simulink model "W01_Base_World_real_time_cs"  (R2019a)
settings: Solver=FixedStepDiscrete  StartTime=0.0  StopTime=100  FixedStep=1/10  RelTol=1e-3
PreLoadFcn:
  | mbxruntime.callbacks.PreLoadFcn(bdroot);
  | check_NUTS_defined
  | model_closed = 0;
  | assignin('base',['model_closed_' bdroot],false);
PostLoadFcn:
  | mbxruntime.callbacks.PostLoadFcn(bdroot);
InitFcn:
  | mbxruntime.callbacks.InitFcn(bdroot);
StartFcn:
  | mbxruntime.callbacks.StartFcn(bdroot);
StopFcn:
  | mbxruntime.callbacks.StopFcn(bdroot);;
  | 
model workspace: external: MAT-File .\W01_Base_World_real_time_cs_hws.mat (data not in the file)
undefined symbols (not defined in the file): DiscIntNeverNeededParam, Header, InitImageOutputDir, mbxruntime, Orientation, Poses, Poses_SL_Info, Position, tabledata, W01_Base_World_real_time_cs_0b088fecc0986594, W01_Base_World_real_time_cs_1aae0b63dd3ae7f4, W01_Base_World_real_time_cs_220fcdeecd830796, W01_Base_World_real_time_cs_3877e8e14bce73ac, W01_Base_World_real_time_cs_4300902b6df2ef4f, W01_Base_World_real_time_cs_4b27c2527ab847ef, W01_Base_World_real_time_cs_5a21cbbf439ca820, W01_Base_World_real_time_cs_5fa564e8c61193e5, W01_Base_World_real_time_cs_830b936d13a49cea, W01_Base_World_real_time_cs_930ade6322553a76, W01_Base_World_real_time_cs_ac8882985e6a0180, W01_Base_World_real_time_cs_ae21d31eb95a5608, W01_Base_World_real_time_cs_Audi_A8_Sedan_1_Path_pathUniqueID, W01_Base_World_real_time_cs_b246a85ce45846f9, W01_Base_World_real_time_cs_b2518551f2cbcab1, W01_Base_World_real_time_cs_b7bc831679541a88, W01_Base_World_real_time_cs_dae62575d56496ac, W01_Base_World_real_time_cs_de41d194e5862055, W01_Base_World_real_time_cs_Male_RegularAni_1_Path_pathUniqueID, W01_Base_World_real_time_cs_Male_RegularAni_2_Path_pathUniqueID
libraries: adeye_lib x37, simulink_extras x30, simulink x10, robotlib x4, sharedtransform x2, PreScanSimulinkLibrary x2
(part 4 of 8)

== system W01_Base_World_real_time_cs/PreScanTerminator ==
  Terminator : Terminator
  sfun_Terminator : S-Function  FunctionName=sfun_Terminator  Parameters=SampleTime  SFunctionDeploymentMode=off  EnableBusSupport=off  mask(Legacy Function){SFunctionSpec=void prescan_terminator_outputFcn(void ** work1, PRESCAN_TERMINATORDATA y1[1]), SampleTime=TimeStep, ShowSpec=on}
      mask prompts: SampleTime "Sample time (-1 for inherited):"; ShowSpec "Display function specification"
      mask help:
      | This block allows you to call the legacy functions specified by the following Legacy Code Tool definition:
      | def.SFunctionName = 'sfun_Terminator';
      | def.OutputFcnSpec = 'void prescan_terminator_outputFcn(void ** work1, PRESCAN_TERMINATORDATA y1[1])';
      | def.StartFcnSpec = 'void prescan_terminator_startFcn(void ** work1)';
      | def.TerminateFcnSpec = 'void prescan_terminator_terminateFcn(void ** work1)';
      | def.HeaderFiles = {'prescan_terminator_data.h'};
      | def.HostLibFiles = {'sensorinterfaced.lib'};
      | def.IncPaths = {'src', 'C:\prescandev\vislibrary\vis\..\pimp\include\sensors\InterfaceRTW'};
      | def.SrcPaths = {'src'};
      | def.LibPaths = {'C:\\prescandev\\vislibrary_build\lib'};
      | def.SampleTime = 'parameterized';
      | def.Options.language = 'C';
      mask Help: <p>This block was generated automatically by the Legacy Code Tool. For detailed help on this tool, call<a href="matlab:legacy_code('help')"> legacy_code('help')</a>.</p>
      mask Callback ShowSpec:
      | if strcmp(get_param(gcbh, 'ShowSpec'), 'on')
      |   set_param(gcbh, 'MaskDisplay', sprintf('fprintf(''%s'');', get_param(gcbh, 'SFunctionSpec')));
      | else
      |   set_param(gcbh, 'MaskDisplay', sprintf('fprintf(''%s'');', get_param(gcbh, 'FunctionName')));
      | end
      mask Display: fprintf('void prescan_terminator_outputFcn(void ** work1, PRESCAN_TERMINATORDATA y1[1])');
  wires:
  sfun_Terminator/1 -> Terminator/1

== system W01_Base_World_real_time_cs/SELF_Audi_A8_Sedan_1 ==
  Sensor : S-Function  FunctionName=sfun_SelfSensor  Parameters=mbxruntime.parameters.convert(UniqueID), mbxruntime.parameters.convert(TimeStep)  SFunctionDeploymentMode=off  EnableBusSupport=off  mask(PreScan Source Block: SELF){UniqueID=18645, TimeStep=1/10}
      mask prompts: UniqueID "Auto-Assigned: Unique ID"; TimeStep "Auto-Assigned: Upload Period [s]"
      mask help:
      | The SELF port shows (state) information of the actor itself. The outputs are position in the experiment's axis system and the GPS coordinates, and the object's absolute velocity and compass heading.
      |
      | For more information, please click Help.
      mask Help: eval('openHelp(462)')
      mask Display: image(imread('GPS.png'))
  SELF_Audi_A8_Sedan_1 : Outport  Tag=outport/SelfPort  OutDataTypeStr=Bus: PRESCAN_SELFSENSORDATA  PortDimensions=1  SampleTime=1/10
  wires:
  Sensor/1 -> SELF_Audi_A8_Sedan_1/1

== system W01_Base_World_real_time_cs/SELF_BMW_X5_SUV_1 ==
  Sensor : S-Function  FunctionName=sfun_SelfSensor  Parameters=mbxruntime.parameters.convert(UniqueID), mbxruntime.parameters.convert(TimeStep)  SFunctionDeploymentMode=off  EnableBusSupport=off  mask(PreScan Source Block: SELF){UniqueID=9040, TimeStep=1/10}
      mask prompts: UniqueID "Auto-Assigned: Unique ID"; TimeStep "Auto-Assigned: Upload Period [s]"
      mask help:
      | The SELF port shows (state) information of the actor itself. The outputs are position in the experiment's axis system and the GPS coordinates, and the object's absolute velocity and compass heading.
      |
      | For more information, please click Help.
      mask Help: eval('openHelp(462)')
      mask Display: image(imread('GPS.png'))
  SELF_BMW_X5_SUV_1 : Outport  Tag=outport/SelfPort  OutDataTypeStr=Bus: PRESCAN_SELFSENSORDATA  PortDimensions=1  SampleTime=1/10
  wires:
  Sensor/1 -> SELF_BMW_X5_SUV_1/1

== system W01_Base_World_real_time_cs/SELF_Child_RegularAni_1 ==
  Sensor : S-Function  FunctionName=sfun_SelfSensor  Parameters=mbxruntime.parameters.convert(UniqueID), mbxruntime.parameters.convert(TimeStep)  SFunctionDeploymentMode=off  EnableBusSupport=off  mask(PreScan Source Block: SELF){UniqueID=18395, TimeStep=1/10}
      mask prompts: UniqueID "Auto-Assigned: Unique ID"; TimeStep "Auto-Assigned: Upload Period [s]"
      mask help:
      | The SELF port shows (state) information of the actor itself. The outputs are position in the experiment's axis system and the GPS coordinates, and the object's absolute velocity and compass heading.
      |
      | For more information, please click Help.
      mask Help: eval('openHelp(462)')
      mask Display: image(imread('GPS.png'))
  SELF_Child_RegularAni_1 : Outport  Tag=outport/SelfPort  OutDataTypeStr=Bus: PRESCAN_SELFSENSORDATA  PortDimensions=1  SampleTime=1/10
  wires:
  Sensor/1 -> SELF_Child_RegularAni_1/1

== system W01_Base_World_real_time_cs/SELF_Child_RegularAni_2 ==
  Sensor : S-Function  FunctionName=sfun_SelfSensor  Parameters=mbxruntime.parameters.convert(UniqueID), mbxruntime.parameters.convert(TimeStep)  SFunctionDeploymentMode=off  EnableBusSupport=off  mask(PreScan Source Block: SELF){UniqueID=18628, TimeStep=1/10}
      mask prompts: UniqueID "Auto-Assigned: Unique ID"; TimeStep "Auto-Assigned: Upload Period [s]"
      mask help:
      | The SELF port shows (state) information of the actor itself. The outputs are position in the experiment's axis system and the GPS coordinates, and the object's absolute velocity and compass heading.
      |
      | For more information, please click Help.
      mask Help: eval('openHelp(462)')
      mask Display: image(imread('GPS.png'))
  SELF_Child_RegularAni_2 : Outport  Tag=outport/SelfPort  OutDataTypeStr=Bus: PRESCAN_SELFSENSORDATA  PortDimensions=1  SampleTime=1/10
  wires:
  Sensor/1 -> SELF_Child_RegularAni_2/1

== system W01_Base_World_real_time_cs/SELF_Citroen_C3_Hatchback_1 ==
  Sensor : S-Function  FunctionName=sfun_SelfSensor  Parameters=mbxruntime.parameters.convert(UniqueID), mbxruntime.parameters.convert(TimeStep)  SFunctionDeploymentMode=off  EnableBusSupport=off  mask(PreScan Source Block: SELF){UniqueID=18857, TimeStep=1/10}
      mask prompts: UniqueID "Auto-Assigned: Unique ID"; TimeStep "Auto-Assigned: Upload Period [s]"
      mask help:
      | The SELF port shows (state) information of the actor itself. The outputs are position in the experiment's axis system and the GPS coordinates, and the object's absolute velocity and compass heading.
      |
      | For more information, please click Help.
      mask Help: eval('openHelp(462)')
      mask Display: image(imread('GPS.png'))
  SELF_Citroen_C3_Hatchback_1 : Outport  Tag=outport/SelfPort  OutDataTypeStr=Bus: PRESCAN_SELFSENSORDATA  PortDimensions=1  SampleTime=1/10
  wires:
  Sensor/1 -> SELF_Citroen_C3_Hatchback_1/1

== system W01_Base_World_real_time_cs/SELF_Female_RegularAni_1 ==
  Sensor : S-Function  FunctionName=sfun_SelfSensor  Parameters=mbxruntime.parameters.convert(UniqueID), mbxruntime.parameters.convert(TimeStep)  SFunctionDeploymentMode=off  EnableBusSupport=off  mask(PreScan Source Block: SELF){UniqueID=18631, TimeStep=1/10}
      mask prompts: UniqueID "Auto-Assigned: Unique ID"; TimeStep "Auto-Assigned: Upload Period [s]"
      mask help:
      | The SELF port shows (state) information of the actor itself. The outputs are position in the experiment's axis system and the GPS coordinates, and the object's absolute velocity and compass heading.
      |
      | For more information, please click Help.
      mask Help: eval('openHelp(462)')
      mask Display: image(imread('GPS.png'))
  SELF_Female_RegularAni_1 : Outport  Tag=outport/SelfPort  OutDataTypeStr=Bus: PRESCAN_SELFSENSORDATA  PortDimensions=1  SampleTime=1/10
  wires:
  Sensor/1 -> SELF_Female_RegularAni_1/1

== system W01_Base_World_real_time_cs/SELF_Male_RegularAni_1 ==
  Sensor : S-Function  FunctionName=sfun_SelfSensor  Parameters=mbxruntime.parameters.convert(UniqueID), mbxruntime.parameters.convert(TimeStep)  SFunctionDeploymentMode=off  EnableBusSupport=off  mask(PreScan Source Block: SELF){UniqueID=18634, TimeStep=1/10}
      mask prompts: UniqueID "Auto-Assigned: Unique ID"; TimeStep "Auto-Assigned: Upload Period [s]"
      mask help:
      | The SELF port shows (state) information of the actor itself. The outputs are position in the experiment's axis system and the GPS coordinates, and the object's absolute velocity and compass heading.
      |
      | For more information, please click Help.
      mask Help: eval('openHelp(462)')
      mask Display: image(imread('GPS.png'))
  SELF_Male_RegularAni_1 : Outport  Tag=outport/SelfPort  OutDataTypeStr=Bus: PRESCAN_SELFSENSORDATA  PortDimensions=1  SampleTime=1/10
  wires:
  Sensor/1 -> SELF_Male_RegularAni_1/1

== system W01_Base_World_real_time_cs/SELF_Male_RegularAni_2 ==
  Sensor : S-Function  FunctionName=sfun_SelfSensor  Parameters=mbxruntime.parameters.convert(UniqueID), mbxruntime.parameters.convert(TimeStep)  SFunctionDeploymentMode=off  EnableBusSupport=off  mask(PreScan Source Block: SELF){UniqueID=18853, TimeStep=1/10}
      mask prompts: UniqueID "Auto-Assigned: Unique ID"; TimeStep "Auto-Assigned: Upload Period [s]"
      mask help:
      | The SELF port shows (state) information of the actor itself. The outputs are position in the experiment's axis system and the GPS coordinates, and the object's absolute velocity and compass heading.
      |
      | For more information, please click Help.
      mask Help: eval('openHelp(462)')
      mask Display: image(imread('GPS.png'))
  SELF_Male_RegularAni_2 : Outport  Tag=outport/SelfPort  OutDataTypeStr=Bus: PRESCAN_SELFSENSORDATA  PortDimensions=1  SampleTime=1/10
  wires:
  Sensor/1 -> SELF_Male_RegularAni_2/1

== system W01_Base_World_real_time_cs/STATE_Audi_A8_Sedan_1_bus ==
  STATE_Audi_A8_Sedan_1_bus : Inport  Tag=inport/StatePort  OutDataTypeStr=Bus: PRESCAN_STATEACTUATORDATA  PortDimensions=1  SampleTime=1/10  BusOutputAsStruct=on
  Actuator : S-Function  FunctionName=sfun_StateActuator  Parameters=mbxruntime.parameters.convert(UniqueID), mbxruntime.parameters.convert(TimeStep)  SFunctionDeploymentMode=off  EnableBusSupport=off  mask(PreScan Sink Block: State){UniqueID=18645, TimeStep=1/10}
      mask prompts: UniqueID "Auto-Assigned: Unique ID"; TimeStep "Auto-Assigned: Upload Period [s]"
      mask help:
      | The Actor State contains a vector signal of size (9x1), containing the following signals:
      |
      | -  Position    	(x,y,z)             	[m]
      | -  Velocity    	(vx,vy,vz)         	[m/s]
      | -  Angles       	(Roll, Pitch, Yaw)	[rad]
      |
      | The Actor state is defined in the global axis system.
      | The state is superponed on the Initial position defined in the GUI.
      |
      | For more information, please click Help.
      mask Help: eval('openHelp(222)')
      mask Display: image(imread('State.png'))
  wires:
  STATE_Audi_A8_Sedan_1_bus/1 -> Actuator/1

== system W01_Base_World_real_time_cs/STATE_BMW_X5_SUV_1_bus ==
  STATE_BMW_X5_SUV_1_bus : Inport  Tag=inport/StatePort  OutDataTypeStr=Bus: PRESCAN_STATEACTUATORDATA  PortDimensions=1  SampleTime=1/10  BusOutputAsStruct=on
  Actuator : S-Function  FunctionName=sfun_StateActuator  Parameters=mbxruntime.parameters.convert(UniqueID), mbxruntime.parameters.convert(TimeStep)  SFunctionDeploymentMode=off  EnableBusSupport=off  mask(PreScan Sink Block: State){UniqueID=9040, TimeStep=1/10}
      mask prompts: UniqueID "Auto-Assigned: Unique ID"; TimeStep "Auto-Assigned: Upload Period [s]"
      mask help:
      | The Actor State contains a vector signal of size (9x1), containing the following signals:
      |
      | -  Position    	(x,y,z)             	[m]
      | -  Velocity    	(vx,vy,vz)         	[m/s]
      | -  Angles       	(Roll, Pitch, Yaw)	[rad]
      |
      | The Actor state is defined in the global axis system.
      | The state is superponed on the Initial position defined in the GUI.
      |
      | For more information, please click Help.
      mask Help: eval('openHelp(222)')
      mask Display: image(imread('State.png'))
  wires:
  STATE_BMW_X5_SUV_1_bus/1 -> Actuator/1

== system W01_Base_World_real_time_cs/STATE_Child_RegularAni_1_bus ==
  STATE_Child_RegularAni_1_bus : Inport  Tag=inport/StatePort  OutDataTypeStr=Bus: PRESCAN_STATEACTUATORDATA  PortDimensions=1  SampleTime=1/10  BusOutputAsStruct=on
  Actuator : S-Function  FunctionName=sfun_StateActuator  Parameters=mbxruntime.parameters.convert(UniqueID), mbxruntime.parameters.convert(TimeStep)  SFunctionDeploymentMode=off  EnableBusSupport=off  mask(PreScan Sink Block: State){UniqueID=18395, TimeStep=1/10}
      mask prompts: UniqueID "Auto-Assigned: Unique ID"; TimeStep "Auto-Assigned: Upload Period [s]"
      mask help:
      | The Actor State contains a vector signal of size (9x1), containing the following signals:
      |
      | -  Position    	(x,y,z)             	[m]
      | -  Velocity    	(vx,vy,vz)         	[m/s]
      | -  Angles       	(Roll, Pitch, Yaw)	[rad]
      |
      | The Actor state is defined in the global axis system.
      | The state is superponed on the Initial position defined in the GUI.
      |
      | For more information, please click Help.
      mask Help: eval('openHelp(222)')
      mask Display: image(imread('State.png'))
  wires:
  STATE_Child_RegularAni_1_bus/1 -> Actuator/1

== system W01_Base_World_real_time_cs/STATE_Child_RegularAni_2_bus ==
  STATE_Child_RegularAni_2_bus : Inport  Tag=inport/StatePort  OutDataTypeStr=Bus: PRESCAN_STATEACTUATORDATA  PortDimensions=1  SampleTime=1/10  BusOutputAsStruct=on
  Actuator : S-Function  FunctionName=sfun_StateActuator  Parameters=mbxruntime.parameters.convert(UniqueID), mbxruntime.parameters.convert(TimeStep)  SFunctionDeploymentMode=off  EnableBusSupport=off  mask(PreScan Sink Block: State){UniqueID=18628, TimeStep=1/10}
      mask prompts: UniqueID "Auto-Assigned: Unique ID"; TimeStep "Auto-Assigned: Upload Period [s]"
      mask help:
      | The Actor State contains a vector signal of size (9x1), containing the following signals:
      |
      | -  Position    	(x,y,z)             	[m]
      | -  Velocity    	(vx,vy,vz)         	[m/s]
      | -  Angles       	(Roll, Pitch, Yaw)	[rad]
      |
      | The Actor state is defined in the global axis system.
      | The state is superponed on the Initial position defined in the GUI.
      |
      | For more information, please click Help.
      mask Help: eval('openHelp(222)')
      mask Display: image(imread('State.png'))
  wires:
  STATE_Child_RegularAni_2_bus/1 -> Actuator/1

== system W01_Base_World_real_time_cs/STATE_Citroen_C3_Hatchback_1_bus ==
  STATE_Citroen_C3_Hatchback_1_bus : Inport  Tag=inport/StatePort  OutDataTypeStr=Bus: PRESCAN_STATEACTUATORDATA  PortDimensions=1  SampleTime=1/10  BusOutputAsStruct=on
  Actuator : S-Function  FunctionName=sfun_StateActuator  Parameters=mbxruntime.parameters.convert(UniqueID), mbxruntime.parameters.convert(TimeStep)  SFunctionDeploymentMode=off  EnableBusSupport=off  mask(PreScan Sink Block: State){UniqueID=18857, TimeStep=1/10}
      mask prompts: UniqueID "Auto-Assigned: Unique ID"; TimeStep "Auto-Assigned: Upload Period [s]"
      mask help:
      | The Actor State contains a vector signal of size (9x1), containing the following signals:
      |
      | -  Position    	(x,y,z)             	[m]
      | -  Velocity    	(vx,vy,vz)         	[m/s]
      | -  Angles       	(Roll, Pitch, Yaw)	[rad]
      |
      | The Actor state is defined in the global axis system.
      | The state is superponed on the Initial position defined in the GUI.
      |
      | For more information, please click Help.
      mask Help: eval('openHelp(222)')
      mask Display: image(imread('State.png'))
  wires:
  STATE_Citroen_C3_Hatchback_1_bus/1 -> Actuator/1

== system W01_Base_World_real_time_cs/STATE_Female_RegularAni_1_bus ==
  STATE_Female_RegularAni_1_bus : Inport  Tag=inport/StatePort  OutDataTypeStr=Bus: PRESCAN_STATEACTUATORDATA  PortDimensions=1  SampleTime=1/10  BusOutputAsStruct=on
  Actuator : S-Function  FunctionName=sfun_StateActuator  Parameters=mbxruntime.parameters.convert(UniqueID), mbxruntime.parameters.convert(TimeStep)  SFunctionDeploymentMode=off  EnableBusSupport=off  mask(PreScan Sink Block: State){UniqueID=18631, TimeStep=1/10}
      mask prompts: UniqueID "Auto-Assigned: Unique ID"; TimeStep "Auto-Assigned: Upload Period [s]"
      mask help:
      | The Actor State contains a vector signal of size (9x1), containing the following signals:
      |
      | -  Position    	(x,y,z)             	[m]
      | -  Velocity    	(vx,vy,vz)         	[m/s]
      | -  Angles       	(Roll, Pitch, Yaw)	[rad]
      |
      | The Actor state is defined in the global axis system.
      | The state is superponed on the Initial position defined in the GUI.
      |
      | For more information, please click Help.
      mask Help: eval('openHelp(222)')
      mask Display: image(imread('State.png'))
  wires:
  STATE_Female_RegularAni_1_bus/1 -> Actuator/1

== system W01_Base_World_real_time_cs/STATE_Male_RegularAni_1_bus ==
  STATE_Male_RegularAni_1_bus : Inport  Tag=inport/StatePort  OutDataTypeStr=Bus: PRESCAN_STATEACTUATORDATA  PortDimensions=1  SampleTime=1/10  BusOutputAsStruct=on
  Actuator : S-Function  FunctionName=sfun_StateActuator  Parameters=mbxruntime.parameters.convert(UniqueID), mbxruntime.parameters.convert(TimeStep)  SFunctionDeploymentMode=off  EnableBusSupport=off  mask(PreScan Sink Block: State){UniqueID=18634, TimeStep=1/10}
      mask prompts: UniqueID "Auto-Assigned: Unique ID"; TimeStep "Auto-Assigned: Upload Period [s]"
      mask help:
      | The Actor State contains a vector signal of size (9x1), containing the following signals:
      |
      | -  Position    	(x,y,z)             	[m]
      | -  Velocity    	(vx,vy,vz)         	[m/s]
      | -  Angles       	(Roll, Pitch, Yaw)	[rad]
      |
      | The Actor state is defined in the global axis system.
      | The state is superponed on the Initial position defined in the GUI.
      |
      | For more information, please click Help.
      mask Help: eval('openHelp(222)')
      mask Display: image(imread('State.png'))
  wires:
  STATE_Male_RegularAni_1_bus/1 -> Actuator/1

== system W01_Base_World_real_time_cs/STATE_Male_RegularAni_2_bus ==
  STATE_Male_RegularAni_2_bus : Inport  Tag=inport/StatePort  OutDataTypeStr=Bus: PRESCAN_STATEACTUATORDATA  PortDimensions=1  SampleTime=1/10  BusOutputAsStruct=on
  Actuator : S-Function  FunctionName=sfun_StateActuator  Parameters=mbxruntime.parameters.convert(UniqueID), mbxruntime.parameters.convert(TimeStep)  SFunctionDeploymentMode=off  EnableBusSupport=off  mask(PreScan Sink Block: State){UniqueID=18853, TimeStep=1/10}
      mask prompts: UniqueID "Auto-Assigned: Unique ID"; TimeStep "Auto-Assigned: Upload Period [s]"
      mask help:
      | The Actor State contains a vector signal of size (9x1), containing the following signals:
      |
      | -  Position    	(x,y,z)             	[m]
      | -  Velocity    	(vx,vy,vz)         	[m/s]
      | -  Angles       	(Roll, Pitch, Yaw)	[rad]
      |
      | The Actor state is defined in the global axis system.
      | The state is superponed on the Initial position defined in the GUI.
      |
      | For more information, please click Help.
      mask Help: eval('openHelp(222)')
      mask Display: image(imread('State.png'))
  wires:
  STATE_Male_RegularAni_2_bus/1 -> Actuator/1

== system W01_Base_World_real_time_cs/ScenarioEngine ==
  Clock : Clock
  sfun_ScenarioEngine : S-Function  FunctionName=sfun_ScenarioEngine  Parameters=TimeStep  SFunctionDeploymentMode=off  EnableBusSupport=off
  wires:
  Clock/1 -> sfun_ScenarioEngine/1

== system W01_Base_World_real_time_cs/Synchronizer ==
  Bus Selector1 : BusSelector  OutputSignals=FederateStopped
  Stop Simulation : Stop
  sfun_Synchronizer : S-Function  FunctionName=sfun_Synchronizer  Parameters=SampleTime  SFunctionDeploymentMode=off  EnableBusSupport=off  mask(Legacy Function){SFunctionSpec=void prescan_synchronizer_outputFcn(void ** work1, PRESCAN_SYNCHRONIZEDATA y1[1]), SampleTime=TimeStep, ShowSpec=on}
      mask prompts: SampleTime "Sample time (-1 for inherited):"; ShowSpec "Display function specification"
      mask help:
      | This block allows you to call the legacy functions specified by the following Legacy Code Tool definition:
      | def.SFunctionName = 'sfun_Synchronizer';
      | def.OutputFcnSpec = 'void prescan_synchronizer_outputFcn(void ** work1, PRESCAN_TIMESTAMPDATA u1[1], PRESCAN_SYNCHRONIZEDATA y1[1])';
      | def.StartFcnSpec = 'void prescan_synchronizer_startFcn(void ** work1)';
      | def.TerminateFcnSpec = 'void prescan_synchronizer_terminateFcn(void ** work1)';
      | def.HeaderFiles = {'prescan_synchronizer_data.h'};
      | def.HostLibFiles = {'sensorinterfaced.lib'};
      | def.IncPaths = {'src', 'C:\prescandev\vislibrary\vis\..\pimp\include\sensors\InterfaceRTW'};
      | def.SrcPaths = {'src'};
      | def.LibPaths = {'C:\\prescandev\\vislibrary_build\lib'};
      | def.SampleTime = 'parameterized';
      | def.Options.language = 'C';
      mask Help: <p>This block was generated automatically by the Legacy Code Tool. For detailed help on this tool, call<a href="matlab:legacy_code('help')"> legacy_code('help')</a>.</p>
      mask Callback ShowSpec:
      | if strcmp(get_param(gcbh, 'ShowSpec'), 'on')
      |   set_param(gcbh, 'MaskDisplay', sprintf('fprintf(''%s'');', get_param(gcbh, 'SFunctionSpec')));
      | else
      |   set_param(gcbh, 'MaskDisplay', sprintf('fprintf(''%s'');', get_param(gcbh, 'FunctionName')));
      | end
      mask Display: fprintf('void prescan_synchronizer_outputFcn(void ** work1, PRESCAN_SYNCHRONIZEDATA y1[1])');
  wires:
  sfun_Synchronizer/1 -> Bus Selector1/1
  Bus Selector1/1 -> Stop Simulation/1  "<FederateStopped>"

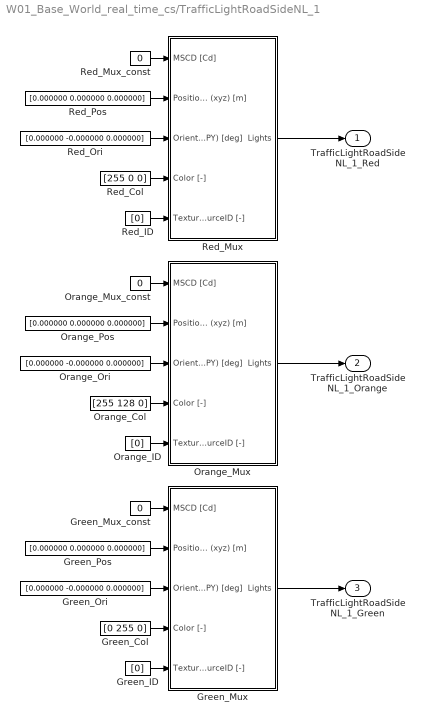
== system W01_Base_World_real_time_cs/TrafficLightRoadSideNL_1 ==
  Green_Col : Constant  Tag=VisuLightConst  Value=[0 255 0]
  Green_ID : Constant  Tag=VisuLightConst  Value=[0]
  Green_Mux : Subsystem  Tag=mux/ActiveLight  mask(PreScan User Interface: VisuActiveLight){}
      mask help:
      | The VisuActiveLight block provides a way for detailed animation of Light Sources, such as the indicator, brake, fog and main lights of a vehicle, or a light post.
      |
      | For more information, please click Help.
      settings: DeleteFcn=PreScanBlockDeleteFcn;
      mask Help: eval('openHelp(209)')
  Green_Mux_const : Constant  Tag=VisuLightConst  Value=0
  Green_Ori : Constant  Tag=VisuLightConst  Value=[0.000000 -0.000000 0.000000]
  Green_Pos : Constant  Tag=VisuLightConst  Value=[0.000000 0.000000 0.000000]
  Orange_Col : Constant  Tag=VisuLightConst  Value=[255 128 0]
  Orange_ID : Constant  Tag=VisuLightConst  Value=[0]
  Orange_Mux : Subsystem  Tag=mux/ActiveLight  mask(PreScan User Interface: VisuActiveLight){}
      mask help:
      | The VisuActiveLight block provides a way for detailed animation of Light Sources, such as the indicator, brake, fog and main lights of a vehicle, or a light post.
      |
      | For more information, please click Help.
      settings: DeleteFcn=PreScanBlockDeleteFcn;
      mask Help: eval('openHelp(209)')
  Orange_Mux_const : Constant  Tag=VisuLightConst  Value=0
  Orange_Ori : Constant  Tag=VisuLightConst  Value=[0.000000 -0.000000 0.000000]
  Orange_Pos : Constant  Tag=VisuLightConst  Value=[0.000000 0.000000 0.000000]
  Red_Col : Constant  Tag=VisuLightConst  Value=[255 0 0]
  Red_ID : Constant  Tag=VisuLightConst  Value=[0]
  Red_Mux : Subsystem  Tag=mux/ActiveLight  mask(PreScan User Interface: VisuActiveLight){}
      mask help:
      | The VisuActiveLight block provides a way for detailed animation of Light Sources, such as the indicator, brake, fog and main lights of a vehicle, or a light post.
      |
      | For more information, please click Help.
      settings: DeleteFcn=PreScanBlockDeleteFcn;
      mask Help: eval('openHelp(209)')
  Red_Mux_const : Constant  Tag=VisuLightConst  Value=0
  Red_Ori : Constant  Tag=VisuLightConst  Value=[0.000000 -0.000000 0.000000]
  Red_Pos : Constant  Tag=VisuLightConst  Value=[0.000000 0.000000 0.000000]
  TrafficLightRoadSideNL_1_Red : Outport  Tag=outport/Red  OutDataTypeStr=Bus: PRESCAN_VISULIGHTACTUATOR_DATA  SampleTime=1/10
  TrafficLightRoadSideNL_1_Orange : Outport  Tag=outport/Orange  Port=2  OutDataTypeStr=Bus: PRESCAN_VISULIGHTACTUATOR_DATA  SampleTime=1/10
  TrafficLightRoadSideNL_1_Green : Outport  Tag=outport/Green  Port=3  OutDataTypeStr=Bus: PRESCAN_VISULIGHTACTUATOR_DATA  SampleTime=1/10
  wires:
  Green_Mux_const/1 -> Green_Mux/1(MSCD [Cd])
  Orange_Mux_const/1 -> Orange_Mux/1(MSCD [Cd])
  Red_Mux_const/1 -> Red_Mux/1(MSCD [Cd])
  Red_Mux/1(Lights) -> TrafficLightRoadSideNL_1_Red/1
  Red_Pos/1 -> Red_Mux/2(Position (xyz) [m])
  Red_Ori/1 -> Red_Mux/3(Orientation (RPY) [deg])
  Red_Col/1 -> Red_Mux/4(Color [-])
  Red_ID/1 -> Red_Mux/5(TextureResourceID [-])
  Orange_Mux/1(Lights) -> TrafficLightRoadSideNL_1_Orange/1
  Orange_Pos/1 -> Orange_Mux/2(Position (xyz) [m])
  Orange_Ori/1 -> Orange_Mux/3(Orientation (RPY) [deg])
  Orange_Col/1 -> Orange_Mux/4(Color [-])
  Orange_ID/1 -> Orange_Mux/5(TextureResourceID [-])
  Green_Mux/1(Lights) -> TrafficLightRoadSideNL_1_Green/1
  Green_Pos/1 -> Green_Mux/2(Position (xyz) [m])
  Green_Ori/1 -> Green_Mux/3(Orientation (RPY) [deg])
  Green_Col/1 -> Green_Mux/4(Color [-])
  Green_ID/1 -> Green_Mux/5(TextureResourceID [-])

== system W01_Base_World_real_time_cs/TrafficLightRoadSideNL_1_Green ==
  TrafficLightRoadSideNL_1_Green : Inport  Tag=inport/Green  OutDataTypeStr=Bus: PRESCAN_VISULIGHTACTUATOR_DATA  SampleTime=1/10  BusOutputAsStruct=on
  Actuator : S-Function  FunctionName=sfun_VisuLightActuator  Parameters=mbxruntime.parameters.convert(UniqueID), mbxruntime.parameters.convert(LightName), mbxruntime.parameters.convert(PivotName), mbxruntime.parameters.convert(TextureResources), mbxruntime.parameters.convert(ColorsObjectName), mbxruntime.parameters.convert(MeshOnColor), mbxruntime.parameters.convert(MeshOffColor), tabledata, TimeStep  SFunctionDeploymentMode=off  EnableBusSupport=off  mask(PreScan Sink Block: VisuActiveLight){UniqueID=646, LightName=TrafficLightRoadSideNL_1.LightActuator_2_Green_ActiveLight, PivotName=TrafficLightRoadSideNL_1.Green, TextureResources={ 'Resources/LightMap/GeneralLight.png'}, ColorsObjectName=TrafficLightRoadSideNL_1.Green, MeshOnColor=[0  100    0  255    0  100    0  255  102  102  102  255    0  510    0  255], MeshOffColor=[0  100    0  255    0  100    0  255  102  102  102  255    0    0    0  255], TimeStep=1/10}
      mask prompts: UniqueID "Parent Unique Identifier"; LightName "Light"; PivotName "Pivot"; TextureResources "Texture Resources"; ColorsObjectName "Light Fixture Color Object"; MeshOnColor "Light Fixture On Color"; MeshOffColor "Light Fixture Off Color"; TimeStep "Simulink time step"
      mask help:
      | The VisuActiveLight block provides a way for detailed animation of Light Sources, such as the indicator, brake, fog and main lights of a vehicle, or a light post.
      |
      | For more information, please click Help.
      mask init:
      | [tabledata] = mbxruntime.parameters.table(UniqueID,LightName,PivotName,TextureResources,ColorsObjectName,MeshOnColor,MeshOffColor);
      mask Help: eval('openHelp(209)')
      mask Display: image(imread('HeadLight.png'))
  wires:
  TrafficLightRoadSideNL_1_Green/1 -> Actuator/1

== system W01_Base_World_real_time_cs/TrafficLightRoadSideNL_1_Orange ==
  TrafficLightRoadSideNL_1_Orange : Inport  Tag=inport/Orange  OutDataTypeStr=Bus: PRESCAN_VISULIGHTACTUATOR_DATA  SampleTime=1/10  BusOutputAsStruct=on
  Actuator : S-Function  FunctionName=sfun_VisuLightActuator  Parameters=mbxruntime.parameters.convert(UniqueID), mbxruntime.parameters.convert(LightName), mbxruntime.parameters.convert(PivotName), mbxruntime.parameters.convert(TextureResources), mbxruntime.parameters.convert(ColorsObjectName), mbxruntime.parameters.convert(MeshOnColor), mbxruntime.parameters.convert(MeshOffColor), tabledata, TimeStep  SFunctionDeploymentMode=off  EnableBusSupport=off  mask(PreScan Sink Block: VisuActiveLight){UniqueID=646, LightName=TrafficLightRoadSideNL_1.LightActuator_1_Orange_ActiveLight, PivotName=TrafficLightRoadSideNL_1.Orange, TextureResources={ 'Resources/LightMap/GeneralLight.png'}, ColorsObjectName=TrafficLightRoadSideNL_1.Orange, MeshOnColor=[100   50    0  255  100   50    0  255  102  102  102  255  510  256    0  255], MeshOffColor=[100   50    0  255  100   50    0  255  102  102  102  255    0    0    0  255], TimeStep=1/10}
      mask prompts: UniqueID "Parent Unique Identifier"; LightName "Light"; PivotName "Pivot"; TextureResources "Texture Resources"; ColorsObjectName "Light Fixture Color Object"; MeshOnColor "Light Fixture On Color"; MeshOffColor "Light Fixture Off Color"; TimeStep "Simulink time step"
      mask help:
      | The VisuActiveLight block provides a way for detailed animation of Light Sources, such as the indicator, brake, fog and main lights of a vehicle, or a light post.
      |
      | For more information, please click Help.
      mask init:
      | [tabledata] = mbxruntime.parameters.table(UniqueID,LightName,PivotName,TextureResources,ColorsObjectName,MeshOnColor,MeshOffColor);
      mask Help: eval('openHelp(209)')
      mask Display: image(imread('HeadLight.png'))
  wires:
  TrafficLightRoadSideNL_1_Orange/1 -> Actuator/1

== system W01_Base_World_real_time_cs/TrafficLightRoadSideNL_1_Red ==
  TrafficLightRoadSideNL_1_Red : Inport  Tag=inport/Red  OutDataTypeStr=Bus: PRESCAN_VISULIGHTACTUATOR_DATA  SampleTime=1/10  BusOutputAsStruct=on
  Actuator : S-Function  FunctionName=sfun_VisuLightActuator  Parameters=mbxruntime.parameters.convert(UniqueID), mbxruntime.parameters.convert(LightName), mbxruntime.parameters.convert(PivotName), mbxruntime.parameters.convert(TextureResources), mbxruntime.parameters.convert(ColorsObjectName), mbxruntime.parameters.convert(MeshOnColor), mbxruntime.parameters.convert(MeshOffColor), tabledata, TimeStep  SFunctionDeploymentMode=off  EnableBusSupport=off  mask(PreScan Sink Block: VisuActiveLight){UniqueID=646, LightName=TrafficLightRoadSideNL_1.LightActuator_0_Red_ActiveLight, PivotName=TrafficLightRoadSideNL_1.Red, TextureResources={ 'Resources/LightMap/GeneralLight.png'}, ColorsObjectName=TrafficLightRoadSideNL_1.Red, MeshOnColor=[100    0    0  255  100    0    0  255  102  102  102  255  510    0    0  255], MeshOffColor=[100    0    0  255  100    0    0  255  102  102  102  255    0    0    0  255], TimeStep=1/10}
      mask prompts: UniqueID "Parent Unique Identifier"; LightName "Light"; PivotName "Pivot"; TextureResources "Texture Resources"; ColorsObjectName "Light Fixture Color Object"; MeshOnColor "Light Fixture On Color"; MeshOffColor "Light Fixture Off Color"; TimeStep "Simulink time step"
      mask help:
      | The VisuActiveLight block provides a way for detailed animation of Light Sources, such as the indicator, brake, fog and main lights of a vehicle, or a light post.
      |
      | For more information, please click Help.
      mask init:
      | [tabledata] = mbxruntime.parameters.table(UniqueID,LightName,PivotName,TextureResources,ColorsObjectName,MeshOnColor,MeshOffColor);
      mask Help: eval('openHelp(209)')
      mask Display: image(imread('HeadLight.png'))
  wires:
  TrafficLightRoadSideNL_1_Red/1 -> Actuator/1

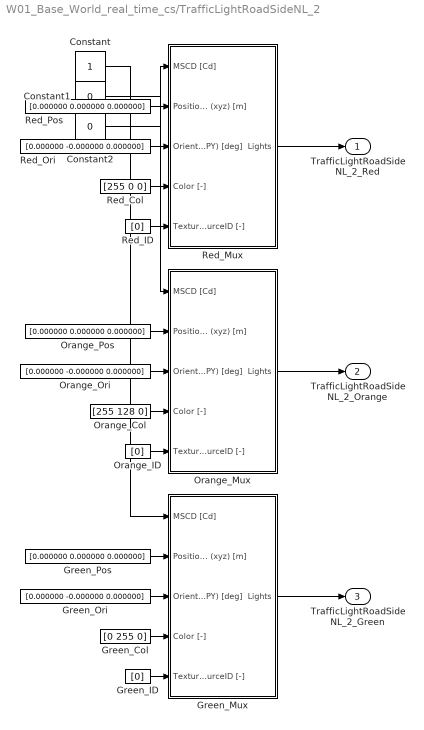
== system W01_Base_World_real_time_cs/TrafficLightRoadSideNL_2 ==
  Constant : Constant
  Constant1 : Constant  Value=0
  Constant2 : Constant  Value=0
  Green_Col : Constant  Tag=VisuLightConst  Value=[0 255 0]
  Green_ID : Constant  Tag=VisuLightConst  Value=[0]
  Green_Mux : Subsystem  Tag=mux/ActiveLight  mask(PreScan User Interface: VisuActiveLight){}
      mask help:
      | The VisuActiveLight block provides a way for detailed animation of Light Sources, such as the indicator, brake, fog and main lights of a vehicle, or a light post.
      |
      | For more information, please click Help.
      settings: DeleteFcn=PreScanBlockDeleteFcn;
      mask Help: eval('openHelp(209)')
  Green_Ori : Constant  Tag=VisuLightConst  Value=[0.000000 -0.000000 0.000000]
  Green_Pos : Constant  Tag=VisuLightConst  Value=[0.000000 0.000000 0.000000]
  Orange_Col : Constant  Tag=VisuLightConst  Value=[255 128 0]
  Orange_ID : Constant  Tag=VisuLightConst  Value=[0]
  Orange_Mux : Subsystem  Tag=mux/ActiveLight  mask(PreScan User Interface: VisuActiveLight){}
      mask help:
      | The VisuActiveLight block provides a way for detailed animation of Light Sources, such as the indicator, brake, fog and main lights of a vehicle, or a light post.
      |
      | For more information, please click Help.
      settings: DeleteFcn=PreScanBlockDeleteFcn;
      mask Help: eval('openHelp(209)')
  Orange_Ori : Constant  Tag=VisuLightConst  Value=[0.000000 -0.000000 0.000000]
  Orange_Pos : Constant  Tag=VisuLightConst  Value=[0.000000 0.000000 0.000000]
  Red_Col : Constant  Tag=VisuLightConst  Value=[255 0 0]
  Red_ID : Constant  Tag=VisuLightConst  Value=[0]
  Red_Mux : Subsystem  Tag=mux/ActiveLight  mask(PreScan User Interface: VisuActiveLight){}
      mask help:
      | The VisuActiveLight block provides a way for detailed animation of Light Sources, such as the indicator, brake, fog and main lights of a vehicle, or a light post.
      |
      | For more information, please click Help.
      settings: DeleteFcn=PreScanBlockDeleteFcn;
      mask Help: eval('openHelp(209)')
  Red_Ori : Constant  Tag=VisuLightConst  Value=[0.000000 -0.000000 0.000000]
  Red_Pos : Constant  Tag=VisuLightConst  Value=[0.000000 0.000000 0.000000]
  TrafficLightRoadSideNL_2_Red : Outport  Tag=outport/Red  OutDataTypeStr=Bus: PRESCAN_VISULIGHTACTUATOR_DATA  SampleTime=1/10
  TrafficLightRoadSideNL_2_Orange : Outport  Tag=outport/Orange  Port=2  OutDataTypeStr=Bus: PRESCAN_VISULIGHTACTUATOR_DATA  SampleTime=1/10
  TrafficLightRoadSideNL_2_Green : Outport  Tag=outport/Green  Port=3  OutDataTypeStr=Bus: PRESCAN_VISULIGHTACTUATOR_DATA  SampleTime=1/10
  wires:
  Constant/1 -> Green_Mux/1(MSCD [Cd])
  Constant1/1 -> Orange_Mux/1(MSCD [Cd])
  Constant2/1 -> Red_Mux/1(MSCD [Cd])
  Red_Mux/1(Lights) -> TrafficLightRoadSideNL_2_Red/1
  Red_Pos/1 -> Red_Mux/2(Position (xyz) [m])
  Red_Ori/1 -> Red_Mux/3(Orientation (RPY) [deg])
  Red_Col/1 -> Red_Mux/4(Color [-])
  Red_ID/1 -> Red_Mux/5(TextureResourceID [-])
  Orange_Mux/1(Lights) -> TrafficLightRoadSideNL_2_Orange/1
  Orange_Pos/1 -> Orange_Mux/2(Position (xyz) [m])
  Orange_Ori/1 -> Orange_Mux/3(Orientation (RPY) [deg])
  Orange_Col/1 -> Orange_Mux/4(Color [-])
  Orange_ID/1 -> Orange_Mux/5(TextureResourceID [-])
  Green_Mux/1(Lights) -> TrafficLightRoadSideNL_2_Green/1
  Green_Pos/1 -> Green_Mux/2(Position (xyz) [m])
  Green_Ori/1 -> Green_Mux/3(Orientation (RPY) [deg])
  Green_Col/1 -> Green_Mux/4(Color [-])
  Green_ID/1 -> Green_Mux/5(TextureResourceID [-])

== system W01_Base_World_real_time_cs/TrafficLightRoadSideNL_2_Green ==
  TrafficLightRoadSideNL_2_Green : Inport  Tag=inport/Green  OutDataTypeStr=Bus: PRESCAN_VISULIGHTACTUATOR_DATA  SampleTime=1/10  BusOutputAsStruct=on
  Actuator : S-Function  FunctionName=sfun_VisuLightActuator  Parameters=mbxruntime.parameters.convert(UniqueID), mbxruntime.parameters.convert(LightName), mbxruntime.parameters.convert(PivotName), mbxruntime.parameters.convert(TextureResources), mbxruntime.parameters.convert(ColorsObjectName), mbxruntime.parameters.convert(MeshOnColor), mbxruntime.parameters.convert(MeshOffColor), tabledata, TimeStep  SFunctionDeploymentMode=off  EnableBusSupport=off  mask(PreScan Sink Block: VisuActiveLight){UniqueID=647, LightName=TrafficLightRoadSideNL_2.LightActuator_2_Green_ActiveLight, PivotName=TrafficLightRoadSideNL_2.Green, TextureResources={ 'Resources/LightMap/GeneralLight.png'}, ColorsObjectName=TrafficLightRoadSideNL_2.Green, MeshOnColor=[0  100    0  255    0  100    0  255  102  102  102  255    0  510    0  255], MeshOffColor=[0  100    0  255    0  100    0  255  102  102  102  255    0    0    0  255], TimeStep=1/10}
      mask prompts: UniqueID "Parent Unique Identifier"; LightName "Light"; PivotName "Pivot"; TextureResources "Texture Resources"; ColorsObjectName "Light Fixture Color Object"; MeshOnColor "Light Fixture On Color"; MeshOffColor "Light Fixture Off Color"; TimeStep "Simulink time step"
      mask help:
      | The VisuActiveLight block provides a way for detailed animation of Light Sources, such as the indicator, brake, fog and main lights of a vehicle, or a light post.
      |
      | For more information, please click Help.
      mask init:
      | [tabledata] = mbxruntime.parameters.table(UniqueID,LightName,PivotName,TextureResources,ColorsObjectName,MeshOnColor,MeshOffColor);
      mask Help: eval('openHelp(209)')
      mask Display: image(imread('HeadLight.png'))
  wires:
  TrafficLightRoadSideNL_2_Green/1 -> Actuator/1

== system W01_Base_World_real_time_cs/TrafficLightRoadSideNL_2_Orange ==
  TrafficLightRoadSideNL_2_Orange : Inport  Tag=inport/Orange  OutDataTypeStr=Bus: PRESCAN_VISULIGHTACTUATOR_DATA  SampleTime=1/10  BusOutputAsStruct=on
  Actuator : S-Function  FunctionName=sfun_VisuLightActuator  Parameters=mbxruntime.parameters.convert(UniqueID), mbxruntime.parameters.convert(LightName), mbxruntime.parameters.convert(PivotName), mbxruntime.parameters.convert(TextureResources), mbxruntime.parameters.convert(ColorsObjectName), mbxruntime.parameters.convert(MeshOnColor), mbxruntime.parameters.convert(MeshOffColor), tabledata, TimeStep  SFunctionDeploymentMode=off  EnableBusSupport=off  mask(PreScan Sink Block: VisuActiveLight){UniqueID=647, LightName=TrafficLightRoadSideNL_2.LightActuator_1_Orange_ActiveLight, PivotName=TrafficLightRoadSideNL_2.Orange, TextureResources={ 'Resources/LightMap/GeneralLight.png'}, ColorsObjectName=TrafficLightRoadSideNL_2.Orange, MeshOnColor=[100   50    0  255  100   50    0  255  102  102  102  255  510  256    0  255], MeshOffColor=[100   50    0  255  100   50    0  255  102  102  102  255    0    0    0  255], TimeStep=1/10}
      mask prompts: UniqueID "Parent Unique Identifier"; LightName "Light"; PivotName "Pivot"; TextureResources "Texture Resources"; ColorsObjectName "Light Fixture Color Object"; MeshOnColor "Light Fixture On Color"; MeshOffColor "Light Fixture Off Color"; TimeStep "Simulink time step"
      mask help:
      | The VisuActiveLight block provides a way for detailed animation of Light Sources, such as the indicator, brake, fog and main lights of a vehicle, or a light post.
      |
      | For more information, please click Help.
      mask init:
      | [tabledata] = mbxruntime.parameters.table(UniqueID,LightName,PivotName,TextureResources,ColorsObjectName,MeshOnColor,MeshOffColor);
      mask Help: eval('openHelp(209)')
      mask Display: image(imread('HeadLight.png'))
  wires:
  TrafficLightRoadSideNL_2_Orange/1 -> Actuator/1

== system W01_Base_World_real_time_cs/TrafficLightRoadSideNL_2_Red ==
  TrafficLightRoadSideNL_2_Red : Inport  Tag=inport/Red  OutDataTypeStr=Bus: PRESCAN_VISULIGHTACTUATOR_DATA  SampleTime=1/10  BusOutputAsStruct=on
  Actuator : S-Function  FunctionName=sfun_VisuLightActuator  Parameters=mbxruntime.parameters.convert(UniqueID), mbxruntime.parameters.convert(LightName), mbxruntime.parameters.convert(PivotName), mbxruntime.parameters.convert(TextureResources), mbxruntime.parameters.convert(ColorsObjectName), mbxruntime.parameters.convert(MeshOnColor), mbxruntime.parameters.convert(MeshOffColor), tabledata, TimeStep  SFunctionDeploymentMode=off  EnableBusSupport=off  mask(PreScan Sink Block: VisuActiveLight){UniqueID=647, LightName=TrafficLightRoadSideNL_2.LightActuator_0_Red_ActiveLight, PivotName=TrafficLightRoadSideNL_2.Red, TextureResources={ 'Resources/LightMap/GeneralLight.png'}, ColorsObjectName=TrafficLightRoadSideNL_2.Red, MeshOnColor=[100    0    0  255  100    0    0  255  102  102  102  255  510    0    0  255], MeshOffColor=[100    0    0  255  100    0    0  255  102  102  102  255    0    0    0  255], TimeStep=1/10}
      mask prompts: UniqueID "Parent Unique Identifier"; LightName "Light"; PivotName "Pivot"; TextureResources "Texture Resources"; ColorsObjectName "Light Fixture Color Object"; MeshOnColor "Light Fixture On Color"; MeshOffColor "Light Fixture Off Color"; TimeStep "Simulink time step"
      mask help:
      | The VisuActiveLight block provides a way for detailed animation of Light Sources, such as the indicator, brake, fog and main lights of a vehicle, or a light post.
      |
      | For more information, please click Help.
      mask init:
      | [tabledata] = mbxruntime.parameters.table(UniqueID,LightName,PivotName,TextureResources,ColorsObjectName,MeshOnColor,MeshOffColor);
      mask Help: eval('openHelp(209)')
      mask Display: image(imread('HeadLight.png'))
  wires:
  TrafficLightRoadSideNL_2_Red/1 -> Actuator/1

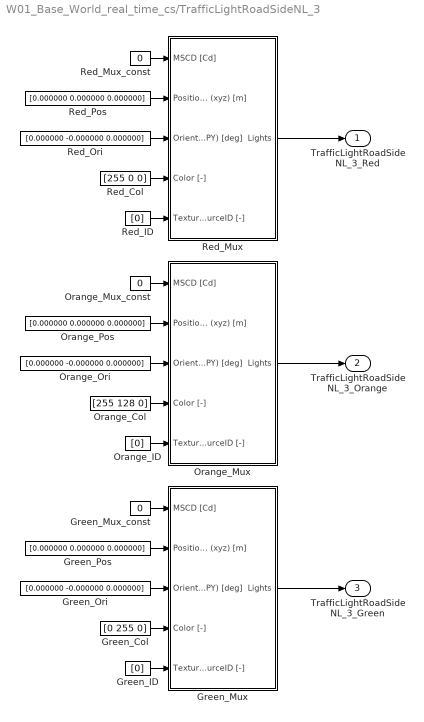
== system W01_Base_World_real_time_cs/TrafficLightRoadSideNL_3 ==
  Green_Col : Constant  Tag=VisuLightConst  Value=[0 255 0]
  Green_ID : Constant  Tag=VisuLightConst  Value=[0]
  Green_Mux : Subsystem  Tag=mux/ActiveLight  mask(PreScan User Interface: VisuActiveLight){}
      mask help:
      | The VisuActiveLight block provides a way for detailed animation of Light Sources, such as the indicator, brake, fog and main lights of a vehicle, or a light post.
      |
      | For more information, please click Help.
      settings: DeleteFcn=PreScanBlockDeleteFcn;
      mask Help: eval('openHelp(209)')
  Green_Mux_const : Constant  Tag=VisuLightConst  Value=0
  Green_Ori : Constant  Tag=VisuLightConst  Value=[0.000000 -0.000000 0.000000]
  Green_Pos : Constant  Tag=VisuLightConst  Value=[0.000000 0.000000 0.000000]
  Orange_Col : Constant  Tag=VisuLightConst  Value=[255 128 0]
  Orange_ID : Constant  Tag=VisuLightConst  Value=[0]
  Orange_Mux : Subsystem  Tag=mux/ActiveLight  mask(PreScan User Interface: VisuActiveLight){}
      mask help:
      | The VisuActiveLight block provides a way for detailed animation of Light Sources, such as the indicator, brake, fog and main lights of a vehicle, or a light post.
      |
      | For more information, please click Help.
      settings: DeleteFcn=PreScanBlockDeleteFcn;
      mask Help: eval('openHelp(209)')
  Orange_Mux_const : Constant  Tag=VisuLightConst  Value=0
  Orange_Ori : Constant  Tag=VisuLightConst  Value=[0.000000 -0.000000 0.000000]
  Orange_Pos : Constant  Tag=VisuLightConst  Value=[0.000000 0.000000 0.000000]
  Red_Col : Constant  Tag=VisuLightConst  Value=[255 0 0]
  Red_ID : Constant  Tag=VisuLightConst  Value=[0]
  Red_Mux : Subsystem  Tag=mux/ActiveLight  mask(PreScan User Interface: VisuActiveLight){}
      mask help:
      | The VisuActiveLight block provides a way for detailed animation of Light Sources, such as the indicator, brake, fog and main lights of a vehicle, or a light post.
      |
      | For more information, please click Help.
      settings: DeleteFcn=PreScanBlockDeleteFcn;
      mask Help: eval('openHelp(209)')
  Red_Mux_const : Constant  Tag=VisuLightConst  Value=0
  Red_Ori : Constant  Tag=VisuLightConst  Value=[0.000000 -0.000000 0.000000]
  Red_Pos : Constant  Tag=VisuLightConst  Value=[0.000000 0.000000 0.000000]
  TrafficLightRoadSideNL_3_Red : Outport  Tag=outport/Red  OutDataTypeStr=Bus: PRESCAN_VISULIGHTACTUATOR_DATA  SampleTime=1/10
  TrafficLightRoadSideNL_3_Orange : Outport  Tag=outport/Orange  Port=2  OutDataTypeStr=Bus: PRESCAN_VISULIGHTACTUATOR_DATA  SampleTime=1/10
  TrafficLightRoadSideNL_3_Green : Outport  Tag=outport/Green  Port=3  OutDataTypeStr=Bus: PRESCAN_VISULIGHTACTUATOR_DATA  SampleTime=1/10
  wires:
  Green_Mux_const/1 -> Green_Mux/1(MSCD [Cd])
  Orange_Mux_const/1 -> Orange_Mux/1(MSCD [Cd])
  Red_Mux_const/1 -> Red_Mux/1(MSCD [Cd])
  Red_Mux/1(Lights) -> TrafficLightRoadSideNL_3_Red/1
  Red_Pos/1 -> Red_Mux/2(Position (xyz) [m])
  Red_Ori/1 -> Red_Mux/3(Orientation (RPY) [deg])
  Red_Col/1 -> Red_Mux/4(Color [-])
  Red_ID/1 -> Red_Mux/5(TextureResourceID [-])
  Orange_Mux/1(Lights) -> TrafficLightRoadSideNL_3_Orange/1
  Orange_Pos/1 -> Orange_Mux/2(Position (xyz) [m])
  Orange_Ori/1 -> Orange_Mux/3(Orientation (RPY) [deg])
  Orange_Col/1 -> Orange_Mux/4(Color [-])
  Orange_ID/1 -> Orange_Mux/5(TextureResourceID [-])
  Green_Mux/1(Lights) -> TrafficLightRoadSideNL_3_Green/1
  Green_Pos/1 -> Green_Mux/2(Position (xyz) [m])
  Green_Ori/1 -> Green_Mux/3(Orientation (RPY) [deg])
  Green_Col/1 -> Green_Mux/4(Color [-])
  Green_ID/1 -> Green_Mux/5(TextureResourceID [-])

== system W01_Base_World_real_time_cs/TrafficLightRoadSideNL_3_Green ==
  TrafficLightRoadSideNL_3_Green : Inport  Tag=inport/Green  OutDataTypeStr=Bus: PRESCAN_VISULIGHTACTUATOR_DATA  SampleTime=1/10  BusOutputAsStruct=on
  Actuator : S-Function  FunctionName=sfun_VisuLightActuator  Parameters=mbxruntime.parameters.convert(UniqueID), mbxruntime.parameters.convert(LightName), mbxruntime.parameters.convert(PivotName), mbxruntime.parameters.convert(TextureResources), mbxruntime.parameters.convert(ColorsObjectName), mbxruntime.parameters.convert(MeshOnColor), mbxruntime.parameters.convert(MeshOffColor), tabledata, TimeStep  SFunctionDeploymentMode=off  EnableBusSupport=off  mask(PreScan Sink Block: VisuActiveLight){UniqueID=649, LightName=TrafficLightRoadSideNL_3.LightActuator_2_Green_ActiveLight, PivotName=TrafficLightRoadSideNL_3.Green, TextureResources={ 'Resources/LightMap/GeneralLight.png'}, ColorsObjectName=TrafficLightRoadSideNL_3.Green, MeshOnColor=[0  100    0  255    0  100    0  255  102  102  102  255    0  510    0  255], MeshOffColor=[0  100    0  255    0  100    0  255  102  102  102  255    0    0    0  255], TimeStep=1/10}
      mask prompts: UniqueID "Parent Unique Identifier"; LightName "Light"; PivotName "Pivot"; TextureResources "Texture Resources"; ColorsObjectName "Light Fixture Color Object"; MeshOnColor "Light Fixture On Color"; MeshOffColor "Light Fixture Off Color"; TimeStep "Simulink time step"
      mask help:
      | The VisuActiveLight block provides a way for detailed animation of Light Sources, such as the indicator, brake, fog and main lights of a vehicle, or a light post.
      |
      | For more information, please click Help.
      mask init:
      | [tabledata] = mbxruntime.parameters.table(UniqueID,LightName,PivotName,TextureResources,ColorsObjectName,MeshOnColor,MeshOffColor);
      mask Help: eval('openHelp(209)')
      mask Display: image(imread('HeadLight.png'))
  wires:
  TrafficLightRoadSideNL_3_Green/1 -> Actuator/1

== system W01_Base_World_real_time_cs/TrafficLightRoadSideNL_3_Orange ==
  TrafficLightRoadSideNL_3_Orange : Inport  Tag=inport/Orange  OutDataTypeStr=Bus: PRESCAN_VISULIGHTACTUATOR_DATA  SampleTime=1/10  BusOutputAsStruct=on
  Actuator : S-Function  FunctionName=sfun_VisuLightActuator  Parameters=mbxruntime.parameters.convert(UniqueID), mbxruntime.parameters.convert(LightName), mbxruntime.parameters.convert(PivotName), mbxruntime.parameters.convert(TextureResources), mbxruntime.parameters.convert(ColorsObjectName), mbxruntime.parameters.convert(MeshOnColor), mbxruntime.parameters.convert(MeshOffColor), tabledata, TimeStep  SFunctionDeploymentMode=off  EnableBusSupport=off  mask(PreScan Sink Block: VisuActiveLight){UniqueID=649, LightName=TrafficLightRoadSideNL_3.LightActuator_1_Orange_ActiveLight, PivotName=TrafficLightRoadSideNL_3.Orange, TextureResources={ 'Resources/LightMap/GeneralLight.png'}, ColorsObjectName=TrafficLightRoadSideNL_3.Orange, MeshOnColor=[100   50    0  255  100   50    0  255  102  102  102  255  510  256    0  255], MeshOffColor=[100   50    0  255  100   50    0  255  102  102  102  255    0    0    0  255], TimeStep=1/10}
      mask prompts: UniqueID "Parent Unique Identifier"; LightName "Light"; PivotName "Pivot"; TextureResources "Texture Resources"; ColorsObjectName "Light Fixture Color Object"; MeshOnColor "Light Fixture On Color"; MeshOffColor "Light Fixture Off Color"; TimeStep "Simulink time step"
      mask help:
      | The VisuActiveLight block provides a way for detailed animation of Light Sources, such as the indicator, brake, fog and main lights of a vehicle, or a light post.
      |
      | For more information, please click Help.
      mask init:
      | [tabledata] = mbxruntime.parameters.table(UniqueID,LightName,PivotName,TextureResources,ColorsObjectName,MeshOnColor,MeshOffColor);
      mask Help: eval('openHelp(209)')
      mask Display: image(imread('HeadLight.png'))
  wires:
  TrafficLightRoadSideNL_3_Orange/1 -> Actuator/1
